simulink model "Map_6_8_s"  (R2023a)
settings: Solver=VariableStepAuto  StartTime=0.0  StopTime=10.0  RelTol=1e-3
undefined symbols (not defined in the file): map_blend_v, map_blend_w, map_lead_den, map_lead_hi_den, map_lead_hi_num, map_lead_num, map_Ta_table, map_Ts_bp, map_v_bp, Ts_ctrl
settings Model: Creator=Tan_Tram  LastModifiedBy=Tan_Tram

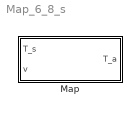
== system Map_6_8_s ==
  Map : Subsystem

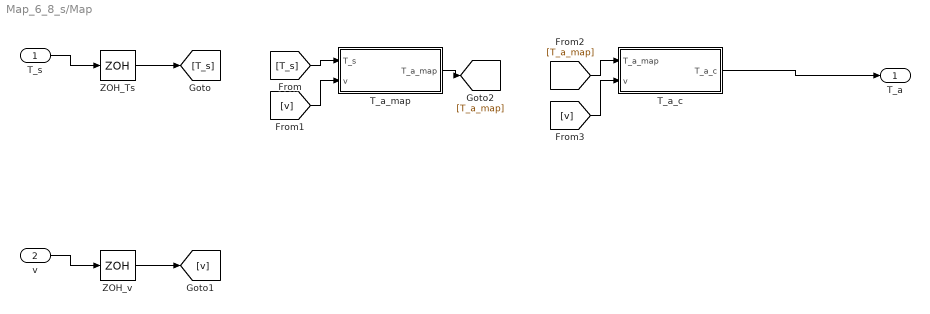
== system Map_6_8_s/Map ==
  T_s : Inport
  v : Inport  Port=2
  T_a_c : Subsystem
  T_a_map : Subsystem
  ZOH_Ts : ZeroOrderHold  SampleTime=Ts_ctrl
  ZOH_v : ZeroOrderHold  SampleTime=Ts_ctrl
  T_a : Outport
  wires:
  T_s/1 -> ZOH_Ts/1
  v/1 -> ZOH_v/1
  ZOH_Ts/1 -> [T_s]
  ZOH_v/1 -> [v]
  [T_s] -> T_a_map/1(T_s)
  [v] -> T_a_map/2(v)
  T_a_map/1(T_a_map) -> [T_a_map]
  [T_a_map] -> T_a_c/1(T_a_map)
  [v] -> T_a_c/2(v)
  T_a_c/1(T_a_c) -> T_a/1

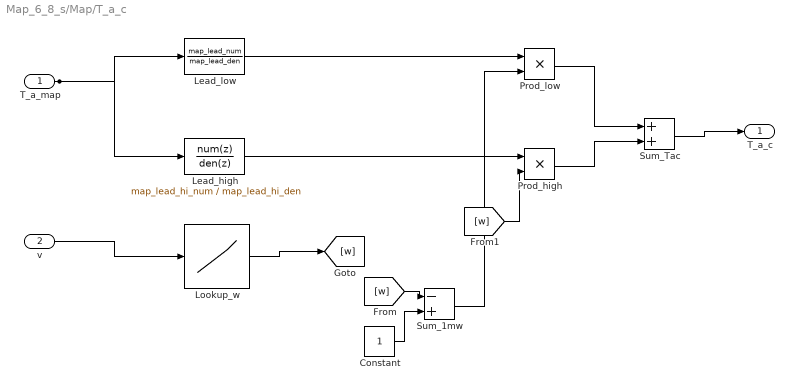
== system Map_6_8_s/Map/T_a_c ==
  T_a_map : Inport
  v : Inport  Port=2
  Constant : Constant
  Lead_high : DiscreteTransferFcn  Numerator=map_lead_hi_num  Denominator=map_lead_hi_den  SampleTime=Ts_ctrl
  Lead_low : DiscreteTransferFcn  Numerator=map_lead_num  Denominator=map_lead_den  SampleTime=Ts_ctrl
  Lookup_w : Lookup_n-D  NumberOfTableDimensions=1  BreakpointsForDimension1=map_blend_v  Table=map_blend_w  ExtrapMethod=Clip  InternalRulePriority=Speed  RndMeth=Simplest
  Prod_high : Product  Inputs=**
  Prod_low : Product  Inputs=**
  Sum_1mw : Sum  Inputs=-+
  Sum_Tac : Sum
  T_a_c : Outport
  wires:
  Lookup_w/1 -> [w]
  Constant/1 -> Sum_1mw/2
  [w] -> Sum_1mw/1
  v/1 -> Lookup_w/1
  T_a_map/1 -> Lead_low/1, Lead_high/1
  Lead_low/1 -> Prod_low/1
  Sum_1mw/1 -> Prod_low/2
  Lead_high/1 -> Prod_high/1
  [w] -> Prod_high/2
  Prod_low/1 -> Sum_Tac/1
  Prod_high/1 -> Sum_Tac/2
  Sum_Tac/1 -> T_a_c/1

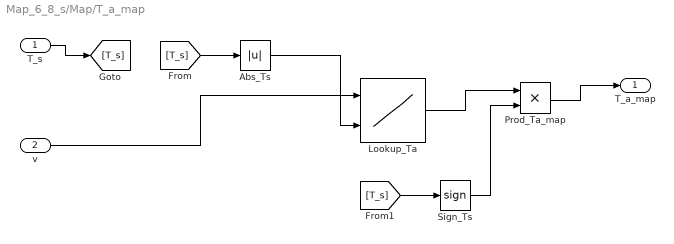
== system Map_6_8_s/Map/T_a_map ==
  T_s : Inport
  v : Inport  Port=2
  Abs_Ts : Abs  SaturateOnIntegerOverflow=off
  Lookup_Ta : Lookup_n-D  BreakpointsForDimension1=map_v_bp  BreakpointsForDimension2=map_Ts_bp  BreakpointsForDimension3=[5, 7]  Table=map_Ta_table  ExtrapMethod=Clip  InternalRulePriority=Speed  RndMeth=Simplest
      settings: InputPortMap=u0,u1
  Prod_Ta_map : Product  Inputs=**
  Sign_Ts : Signum
  T_a_map : Outport
  wires:
  T_s/1 -> [T_s]
  [T_s] -> Abs_Ts/1
  v/1 -> Lookup_Ta/1
  Abs_Ts/1 -> Lookup_Ta/2
  [T_s] -> Sign_Ts/1
  Lookup_Ta/1 -> Prod_Ta_map/1
  Sign_Ts/1 -> Prod_Ta_map/2
  Prod_Ta_map/1 -> T_a_map/1
